simulink model "MRAC"  (R2018a)
settings: Solver=VariableStepAuto  StartTime=0.0  StopTime=10000  FixedStep=0.01  RelTol=1e-3
model workspace (MAT data in the model file):
  A_model = [-7  -14  -8; 1  0  0; 0  1  0]
  A_unknown = [-7.5  -16  -8.5; 1  0  0; 0  1  0]
  B_model = [1; 0; 0]
  B_unknown = [2; 0; 0]
  C_model = [-7 -9 2]
  C_unknown = [-7 -9 2]
  D_model = 0
  D_unknown = 0
  Gamma_r = 1
  Gamma_x = [1  0  0; 0  1  0; 0  0  1]
  K_r_hat_0 = 0
  K_x_hat_0 = [0; 0; 0]
  Lambda = 1
  P = [1  0  0; 0  1  0; 0  0  1]
libraries: cstblocks x2
settings Model: Creator=omery  LastModifiedBy=omery

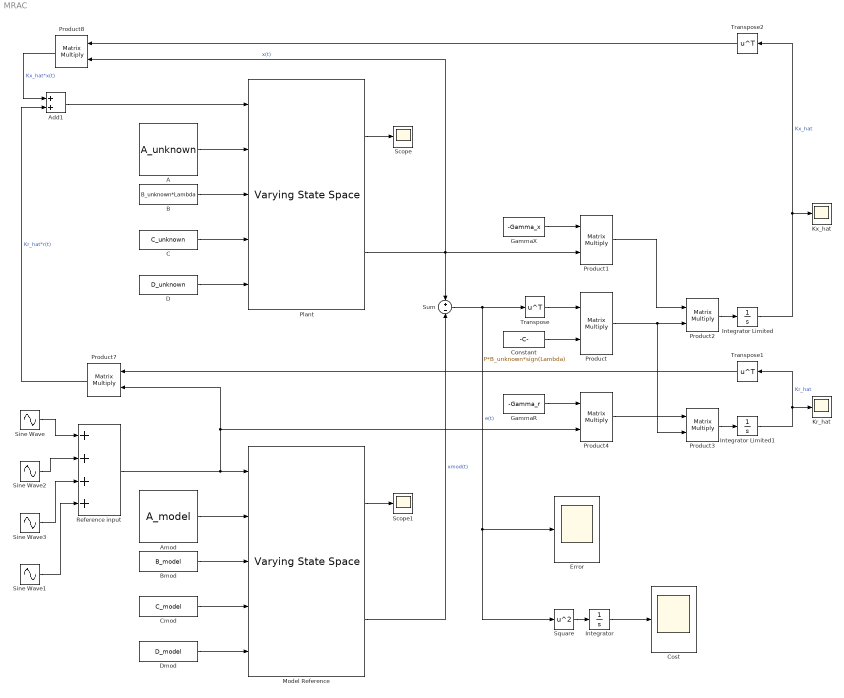
== system MRAC ==
  A : Constant  Value=A_unknown  VectorParams1D=off
  Add1 : Sum
  Amod : Constant  Value=A_model  VectorParams1D=off
  B : Constant  Value=B_unknown*Lambda  VectorParams1D=off
  Bmod : Constant  Value=B_model  VectorParams1D=off
  C : Constant  Value=C_unknown  VectorParams1D=off
  Cmod : Constant  Value=C_model  VectorParams1D=off
  Constant : Constant  Value=P*B_unknown*sign(Lambda)
  Cost : Scope
  D : Constant  Value=D_unknown
  Dmod : Constant  Value=D_model
  Error : Scope
  GammaR : Constant  Value=-Gamma_r
  GammaX : Constant  Value=-Gamma_x
  Integrator : Integrator
  Integrator Limited : Integrator  InitialCondition=K_x_hat_0  LimitOutput=on  UpperSaturationLimit=1  LowerSaturationLimit=0
  Integrator Limited1 : Integrator  InitialCondition=K_r_hat_0  LimitOutput=on  UpperSaturationLimit=1  LowerSaturationLimit=0
  Kr_hat : Scope
  Kx_hat : Scope
  Model Reference : cstblocks/Linear Parameter Varying/Varying State Space  x0=0  xNames=''  OutputX=on  OutputDX=off
      settings: SourceProductName=Control System Toolbox
  Plant : cstblocks/Linear Parameter Varying/Varying State Space  x0=0  xNames=''  OutputX=on  OutputDX=off
      settings: SourceProductName=Control System Toolbox
  Product : Product  SCDEnableBlockLinearizationSpecification=on  Multiplication=Matrix(*)  InputSameDT=on
  Product{1..4,7..8} (6 alike) : Product  SCDEnableBlockLinearizationSpecification=on  Multiplication=Matrix(*)
  Reference input : Sum  Inputs=++++
  Scope : Scope
  Scope1 : Scope
  Sine Wave : Sin  Amplitude=3.5  Frequency=3.5  SampleTime=0
  Sine Wave1 : Sin  SampleTime=0
  Sine Wave2 : Sin  Amplitude=2  Frequency=4  SampleTime=0
  Sine Wave3 : Sin  Amplitude=0.3  Frequency=0.7  SampleTime=0
  Square : Math  Operator=square  SaturateOnIntegerOverflow=on
  Sum : Sum  Inputs=+|-
  Transpose : Math  Operator=transpose  SaturateOnIntegerOverflow=on
  Transpose1 : Math  Operator=transpose  SaturateOnIntegerOverflow=on
  Transpose2 : Math  Operator=transpose  SaturateOnIntegerOverflow=on
  wires:
  Transpose1/1 -> Product7/1
  Product1/1 -> Product2/1
  Transpose/1 -> Product/1
  Sum/1 -> Transpose/1, Error/1, Square/1  "e(t)"
  Add1/1 -> Plant/1
  GammaR/1 -> Product4/1
  Product8/1 -> Add1/1  "Kx_hat*x(t)"
  Product4/1 -> Product3/1
  Product3/1 -> Integrator Limited1/1
  Plant/2 -> Product1/2, Product8/2, Sum/1  "x(t)"
  Product2/1 -> Integrator Limited/1
  Constant/1 -> Product/2
  Cmod/1 -> Model Reference/4
  C/1 -> Plant/4
  Dmod/1 -> Model Reference/5
  Model Reference/2 -> Sum/2  "xmod(t)"
  Integrator Limited/1 -> Transpose2/1, Kx_hat/1  "Kx_hat"
  Plant/1 -> Scope/1
  Transpose2/1 -> Product8/1
  Bmod/1 -> Model Reference/3
  Amod/1 -> Model Reference/2
  D/1 -> Plant/5
  Model Reference/1 -> Scope1/1
  Integrator Limited1/1 -> Kr_hat/1, Transpose1/1  "Kr_hat"
  Product7/1 -> Add1/2  "Kr_hat*r(t)"
  Product/1 -> Product3/2, Product2/2
  GammaX/1 -> Product1/1
  Reference input/1 -> Model Reference/1, Product4/2, Product7/2
  A/1 -> Plant/2
  B/1 -> Plant/3
  Square/1 -> Integrator/1
  Integrator/1 -> Cost/1
  Sine Wave2/1 -> Reference input/2
  Sine Wave/1 -> Reference input/1
  Sine Wave3/1 -> Reference input/3
  Sine Wave1/1 -> Reference input/4
